simulink model "pulse_detector_v2"  (R2022b)
settings: Solver=FixedStepDiscrete  StartTime=0.0  StopTime=SimTime  RelTol=1e-3
undefined symbols (not defined in the file): CorrFilter, threshold, WindowLen
libraries: dspsrcs4 x2, dsphdlfiltering2 x1, simulink x1, hdlsllib x1
settings Model: DataTypeOverride=Off  Creator=Lenovo  LastModifiedBy=Lenovo
settings OptimizationCC: BlockReduction=off  ConditionallyExecuteInputs=off  DefaultParameterBehavior=Inlined  InheritOutputTypeSmallerThanSingle=on
settings DebuggingCC: AlgebraicLoopMsg=error  SingleTaskRateTransMsg=error
settings HardwareCC: ProdBitPerPointer=32  ProdBitPerSizeT=32  ProdBitPerPtrDiffT=32  ProdLargestAtomicFloat=None  ProdIntDivRoundTo=Undefined  ProdEndianess=Unspecified  ProdWordSize=32  ProdHWDeviceType=ASIC/FPGA->ASIC/FPGA  TargetBitPerPointer=64  TargetBitPerSizeT=64  TargetBitPerPtrDiffT=64  TargetLongLongMode=on  TargetIntDivRoundTo=Zero  TargetEndianess=LittleEndian  TargetWordSize=64  TargetHWDeviceType=Custom Processor->MATLAB Host Computer  ProdEqTarget=off

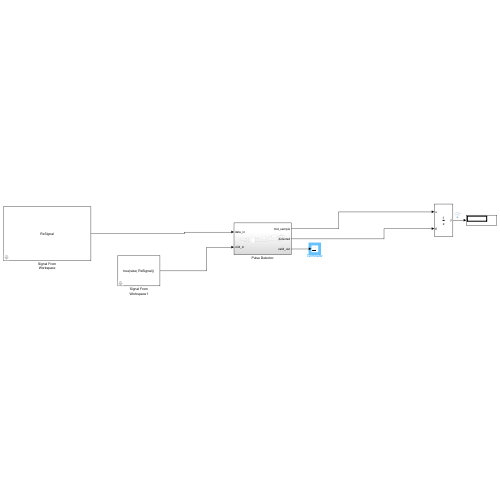
[thumbnail: Simulink's stored preview of the top-level diagram]
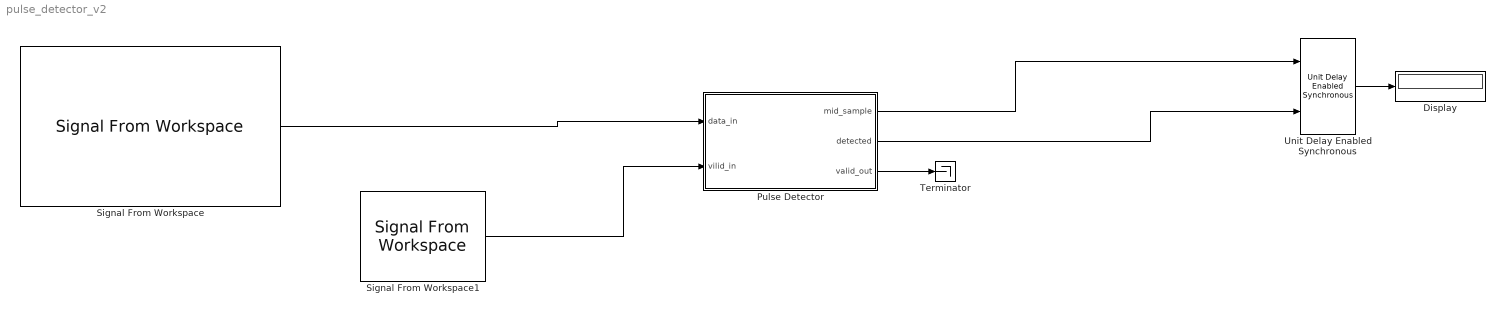
== system pulse_detector_v2 ==
  Display : Display
  Pulse Detector : Subsystem
  Signal From Workspace : dspsrcs4/Signal From Workspace  X=RxSignal  Ts=1  nsamps=1  OutputAfterFinalValue=Setting to zero  ignoreOrWarnInputAndFrameLengths=off  OutputFrames=off
  Signal From Workspace1 : dspsrcs4/Signal From Workspace  X=true(size( RxSignal))  Ts=1  nsamps=1  OutputAfterFinalValue=Setting to zero  ignoreOrWarnInputAndFrameLengths=off  OutputFrames=off
  Terminator : Terminator
  Unit Delay Enabled Synchronous : hdlsllib/Discrete/Unit Delay Enabled Synchronous  InitialCondition=0.0  SampleTime=-1
  wires:
  Unit Delay Enabled Synchronous/1 -> Display/1
  Signal From Workspace/1 -> Pulse Detector/1(data_in)
  Pulse Detector/1(mid_sample) -> Unit Delay Enabled Synchronous/1
  Pulse Detector/2(detected) -> Unit Delay Enabled Synchronous/2
  Signal From Workspace1/1 -> Pulse Detector/2(vilid_in)
  Pulse Detector/3(valid_out) -> Terminator/1

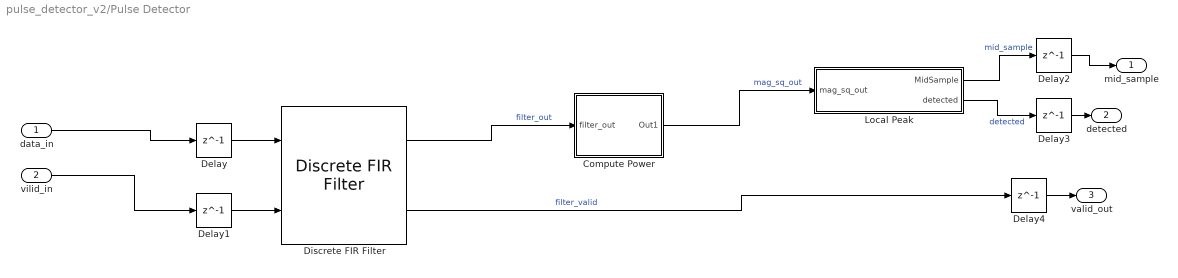
== system pulse_detector_v2/Pulse Detector ==
  data_in : Inport
  vilid_in : Inport  Port=2
  Compute Power : Subsystem
  Delay{,1..4} (5 alike) : Delay  DelayLength=1
  Discrete FIR Filter : dsphdlfiltering2/Discrete FIR Filter  NumeratorSource=Property  Numerator=CorrFilter  NumeratorPrototype=[]  FilterStructure=Direct form systolic  SerializationOption=Minimum number of cycles between valid input samples  NumCycles=2  NumberOfMultipliers=2  SimulateUsing=Code generation  roundingMode=Floor  overflowMode=off  CoefficientsDataTypeStr=Inherit: Same word length as input  ResetInputPort=off  HDLGlobalReset=off
  Local Peak : Subsystem
  mid_sample : Outport
  detected : Outport  Port=2
  valid_out : Outport  Port=3
  wires:
  data_in/1 -> Delay/1
  Compute Power/1(Out1) -> Local Peak/1(mag_sq_out)  "mag_sq_out"
  Discrete FIR Filter/1 -> Compute Power/1(filter_out)  "filter_out"
  Local Peak/1(MidSample) -> Delay2/1  "mid_sample"
  Local Peak/2(detected) -> Delay3/1  "detected"
  vilid_in/1 -> Delay1/1
  Discrete FIR Filter/2 -> Delay4/1  "filter_valid"
  Delay/1 -> Discrete FIR Filter/1
  Delay1/1 -> Discrete FIR Filter/2
  Delay2/1 -> mid_sample/1
  Delay3/1 -> detected/1
  Delay4/1 -> valid_out/1

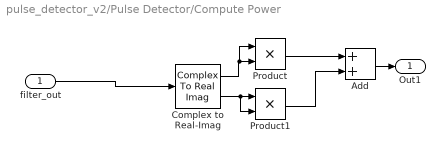
== system pulse_detector_v2/Pulse Detector/Compute Power ==
  filter_out : Inport
  Add : Sum
  Complex to Real-Imag : ComplexToRealImag
  Product : Product
  Product1 : Product
  Out1 : Outport
  wires:
  filter_out/1 -> Complex to Real-Imag/1
  Product/1 -> Add/1
  Complex to Real-Imag/2 -> Product1/2, Product1/1
  Complex to Real-Imag/1 -> Product/1, Product/2
  Product1/1 -> Add/2
  Add/1 -> Out1/1

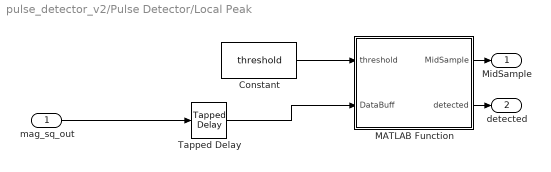
== system pulse_detector_v2/Pulse Detector/Local Peak ==
  mag_sq_out : Inport
  Constant : Constant  Value=threshold
  MATLAB Function : MATLAB Function  TreatAsAtomicUnit=on
  Tapped Delay : simulink/Discrete/Tapped Delay  vinit=0.0  samptime=-1  NumDelays=WindowLen  DelayOrder=Oldest  includeCurrent=off
  MidSample : Outport
  detected : Outport  Port=2
  wires:
  Constant/1 -> MATLAB Function/1(threshold)
  MATLAB Function/2(detected) -> detected/1
  Tapped Delay/1 -> MATLAB Function/2(DataBuff)
  MATLAB Function/1(MidSample) -> MidSample/1
  mag_sq_out/1 -> Tapped Delay/1

== matlab function pulse_detector_v2/Pulse Detector/Local Peak/MATLAB Function ==
  data: MidSample output; threshold input; DataBuff input; detected output; WindowLen parameter
function [MidSample,detected]=fcn(threshold,DataBuff, WindowLen)

MidIdx = ceil(WindowLen/2);

MidSample=DataBuff(MidIdx);
CompareOut=DataBuff-MidSample;



    % if all values in the result are negative and the middle sample is
    % greater than a threshold, it is a local max
if all(CompareOut <= 0) && (MidSample > threshold)
    detected=1;
else
    detected=0;
end
